simulink model "C172S_AltitudeHold_V1"  (R2026a)
settings: Solver=ode4  StartTime=0  StopTime=180  FixedStep=0.02
InitFcn:
  | ah1Data = c172sLongitudinalData();
  | [~,ah1Plant] = c172sLongitudinalPlant(ah1Data);
  | ah1PitchController = c172sPitchAttitudeControllerData();
  | ah1Actuator = c172sElevatorActuatorData();
  | ah1AltitudeController = c172sAltitudeHoldControllerData();
  | A_ah1 = ah1Plant.A; B_ah1 = ah1Plant.B;
  | C_ah1 = ah1Plant.C; D_ah1 = ah1Plant.D;
  | Vtrim_ah1_mps = ah1Data.trim.V_mps;
  | Kh_ah1_per_s = ah1AltitudeController.altitudeGain_per_s;
  | Kv_ah1_radPerMps = ah1AltitudeController.verticalSpeedGain_radPerMps;
  | tauAltitude_ah1_s = ah1AltitudeController.commandFilterTimeConstant_s;
  | hDotLimit_ah1_mps = ah1AltitudeController.verticalSpeedCommandLimit_mps;
  | thetaLimit_ah1_rad = ah1AltitudeController.pitchCommandLimit_rad;
  | Kp_ah1 = ah1PitchController.Kp_radPerRad;
  | Ki_ah1_per_s = ah1PitchController.Ki_radPerRadPerS;
  | Kq_ah1_s = ah1Actuator.integration.Kq_s;
  | tauTheta_ah1_s = ah1PitchController.commandFilterTimeConstant_s;
  | tauActuator_ah1_s = ah1Actuator.dynamics.timeConstant_s;
  | Tt_ah1_s = ah1Actuator.antiWindup.trackingTimeConstant_s;
  | deltaELower_ah1_rad = ah1Actuator.authority.lowerLimit_rad;
  | deltaEUpper_ah1_rad = ah1Actuator.authority.upperLimit_rad;
  | deltaERate_ah1_radps = deg2rad(ah1Actuator.dynamics.rateLimit_degps);
  | if ~exist('hCommand_ah1_m','var'), hCommand_ah1_m = ah1AltitudeController.validation.operationalCommand_m; end
  | if ~exist('antiWindupEnable_ah1','var'), antiWindupEnable_ah1 = 1.0; end
  | if ~exist('x0_ah1','var'), x0_ah1 = zeros(4,1); end
  | if ~exist('xi0_ah1','var'), xi0_ah1 = 0.0; end
  | if ~exist('deltaE0_ah1','var'), deltaE0_ah1 = 0.0; end
  | if ~exist('h0_ah1_m','var'), h0_ah1_m = 0.0; end
undefined symbols (not defined in the file or in its folder): antiWindupEnable_ah1, deltaE0_ah1, h0_ah1_m, x0_ah1, xi0_ah1
settings Model: Creator=Shahi  LastModifiedBy=Shahi

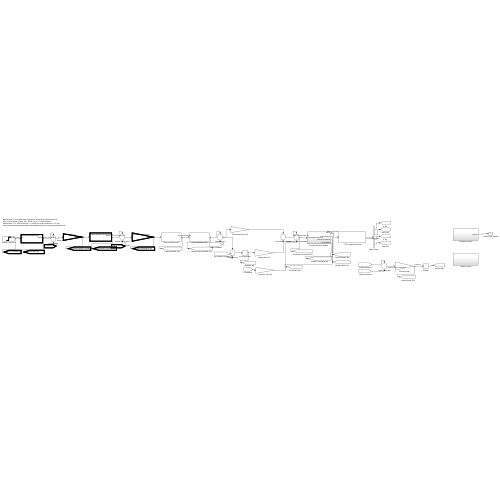
[thumbnail: Simulink's stored preview of the top-level diagram]
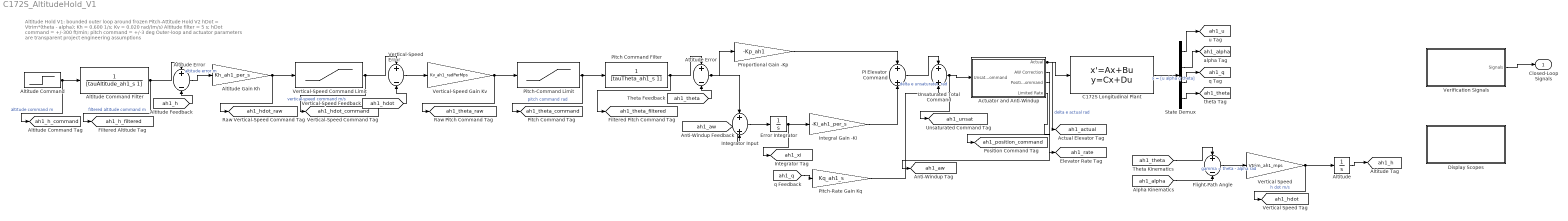
== system C172S_AltitudeHold_V1 ==
  note: Altitude Hold V1: bounded outer loop around frozen Pitch-Attitude Hold V2
      | hDot = Vtrim*(theta - alpha); Kh = 0.600 1/s; Kv = 0.020 rad/(m/s)
      | Altitude filter = 5 s; hDot command = +/-300 ft/min; pitch command = +/-3 deg
      | Outer-loop and actuator parameters are transparent project engineering assumptions
  Actuator and Anti-Windup : Subsystem
  Altitude : Integrator  InitialCondition=h0_ah1_m
  Altitude Command : Step  Time=0  FinalValue=hCommand_ah1_m  SampleTime=0
  Altitude Command Filter : TransferFcn  Numerator=1  Denominator=[tauAltitude_ah1_s 1]
  Altitude Error : Sum  Inputs=+-
  Altitude Gain Kh : Gain  Gain=Kh_ah1_per_s
  Attitude Error : Sum  Inputs=+-
  C172S Longitudinal Plant : StateSpace  A=A_ah1  B=B_ah1  C=C_ah1  D=D_ah1  InitialCondition=x0_ah1
  Display Scopes : Subsystem
  Error Integrator : Integrator  InitialCondition=xi0_ah1
  Flight-Path Angle : Sum  Inputs=+-
  Integral Gain -Ki : Gain  Gain=-Ki_ah1_per_s
  Integrator Input : Sum
  PI Elevator Command : Sum
  Pitch Command Filter : TransferFcn  Numerator=1  Denominator=[tauTheta_ah1_s 1]
  Pitch-Command Limit : Saturate  UpperLimit=thetaLimit_ah1_rad  LowerLimit=-thetaLimit_ah1_rad
  Pitch-Rate Gain Kq : Gain  Gain=Kq_ah1_s
  Proportional Gain -Kp : Gain  Gain=-Kp_ah1
  State Demux : Demux
  Unsaturated Total Command : Sum
  Verification Signals : Subsystem
  Vertical Speed : Gain  Gain=Vtrim_ah1_mps
  Vertical-Speed Command Limit : Saturate  UpperLimit=hDotLimit_ah1_mps  LowerLimit=-hDotLimit_ah1_mps
  Vertical-Speed Error : Sum  Inputs=+-
  Vertical-Speed Gain Kv : Gain  Gain=Kv_ah1_radPerMps
  Closed-Loop Signals : Outport
  tag scope: ah1_actual=global, ah1_alpha=global, ah1_aw=global, ah1_h=global, ah1_h_command=global, ah1_h_filtered=global, ah1_hdot=global, ah1_hdot_command=global, ah1_hdot_raw=global, ah1_position_command=global, ah1_q=global, ah1_rate=global, ah1_theta=global, ah1_theta_command=global, ah1_theta_filtered=global, ah1_theta_raw=global, ah1_u=global, ah1_unsat=global, ah1_xi=global
  wires:
  Altitude Command/1 -> Altitude Command Filter/1, [ah1_h_command]  "altitude command m"
  Altitude Command Filter/1 -> Altitude Error/1, [ah1_h_filtered]  "filtered altitude command m"
  [ah1_h] -> Altitude Error/2
  Altitude Error/1 -> Altitude Gain Kh/1  "altitude error m"
  Altitude Gain Kh/1 -> Vertical-Speed Command Limit/1, [ah1_hdot_raw]
  Vertical-Speed Command Limit/1 -> Vertical-Speed Error/1, [ah1_hdot_command]  "vertical-speed command m/s"
  [ah1_hdot] -> Vertical-Speed Error/2
  Vertical-Speed Error/1 -> Vertical-Speed Gain Kv/1
  Vertical-Speed Gain Kv/1 -> Pitch-Command Limit/1, [ah1_theta_raw]
  Pitch-Command Limit/1 -> Pitch Command Filter/1, [ah1_theta_command]  "pitch command rad"
  Pitch Command Filter/1 -> Attitude Error/1, [ah1_theta_filtered]
  [ah1_theta] -> Attitude Error/2
  Attitude Error/1 -> Proportional Gain -Kp/1, Integrator Input/1
  [ah1_aw] -> Integrator Input/2
  Integrator Input/1 -> Error Integrator/1
  Error Integrator/1 -> Integral Gain -Ki/1, [ah1_xi]
  Proportional Gain -Kp/1 -> PI Elevator Command/1
  Integral Gain -Ki/1 -> PI Elevator Command/2
  [ah1_q] -> Pitch-Rate Gain Kq/1
  PI Elevator Command/1 -> Unsaturated Total Command/1
  Pitch-Rate Gain Kq/1 -> Unsaturated Total Command/2
  Unsaturated Total Command/1 -> Actuator and Anti-Windup/1(Unsaturated Command), [ah1_unsat]  "delta e unsaturated rad"
  Actuator and Anti-Windup/1(Actual) -> C172S Longitudinal Plant/1, [ah1_actual]  "delta e actual rad"
  C172S Longitudinal Plant/1 -> State Demux/1  "x = [u alpha q theta]"
  [ah1_theta] -> Flight-Path Angle/1
  [ah1_alpha] -> Flight-Path Angle/2
  Flight-Path Angle/1 -> Vertical Speed/1  "gamma = theta - alpha rad"
  Vertical Speed/1 -> Altitude/1, [ah1_hdot]  "h dot m/s"
  Actuator and Anti-Windup/2(AW Correction) -> [ah1_aw]
  Actuator and Anti-Windup/3(Position Command) -> [ah1_position_command]
  Actuator and Anti-Windup/4(Limited Rate) -> [ah1_rate]
  Altitude/1 -> [ah1_h]
  State Demux/1 -> [ah1_u]
  State Demux/2 -> [ah1_alpha]
  State Demux/3 -> [ah1_q]
  State Demux/4 -> [ah1_theta]
  Verification Signals/1(Signals) -> Closed-Loop Signals/1

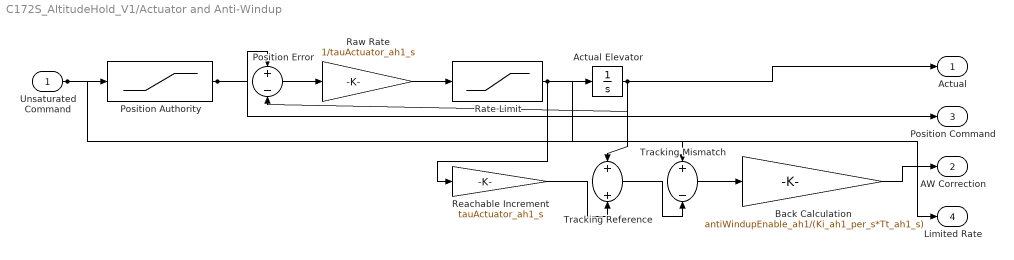
== system C172S_AltitudeHold_V1/Actuator and Anti-Windup ==
  Unsaturated Command : Inport
  Actual Elevator : Integrator  InitialCondition=deltaE0_ah1
  Back Calculation : Gain  Gain=antiWindupEnable_ah1/(Ki_ah1_per_s*Tt_ah1_s)
  Position Authority : Saturate  UpperLimit=deltaEUpper_ah1_rad  LowerLimit=deltaELower_ah1_rad
  Position Error : Sum  Inputs=+-
  Rate Limit : Saturate  UpperLimit=deltaERate_ah1_radps  LowerLimit=-deltaERate_ah1_radps
  Raw Rate : Gain  Gain=1/tauActuator_ah1_s
  Reachable Increment : Gain  Gain=tauActuator_ah1_s
  Tracking Mismatch : Sum  Inputs=+-
  Tracking Reference : Sum
  Actual : Outport
  AW Correction : Outport  Port=2
  Position Command : Outport  Port=3
  Limited Rate : Outport  Port=4
  wires:
  Unsaturated Command/1 -> Position Authority/1, Tracking Mismatch/1
  Position Authority/1 -> Position Error/1, Position Command/1
  Position Error/1 -> Raw Rate/1
  Raw Rate/1 -> Rate Limit/1
  Rate Limit/1 -> Actual Elevator/1, Reachable Increment/1, Limited Rate/1
  Actual Elevator/1 -> Position Error/2, Tracking Reference/1, Actual/1
  Reachable Increment/1 -> Tracking Reference/2
  Tracking Reference/1 -> Tracking Mismatch/2
  Tracking Mismatch/1 -> Back Calculation/1
  Back Calculation/1 -> AW Correction/1

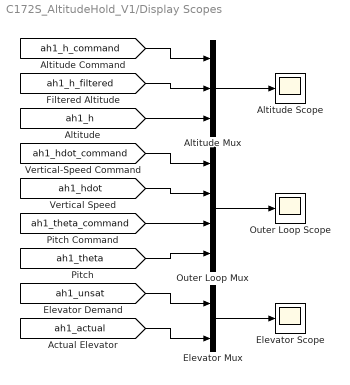
== system C172S_AltitudeHold_V1/Display Scopes ==
  Altitude Mux : Mux  Inputs=3
  Altitude Scope : Scope
  Elevator Mux : Mux  Inputs=2
  Elevator Scope : Scope
  Outer Loop Mux : Mux
  Outer Loop Scope : Scope
  wires:
  [ah1_h_command] -> Altitude Mux/1
  [ah1_h_filtered] -> Altitude Mux/2
  [ah1_h] -> Altitude Mux/3
  Altitude Mux/1 -> Altitude Scope/1
  [ah1_hdot_command] -> Outer Loop Mux/1
  [ah1_hdot] -> Outer Loop Mux/2
  [ah1_theta_command] -> Outer Loop Mux/3
  [ah1_theta] -> Outer Loop Mux/4
  Outer Loop Mux/1 -> Outer Loop Scope/1
  [ah1_unsat] -> Elevator Mux/1
  [ah1_actual] -> Elevator Mux/2
  Elevator Mux/1 -> Elevator Scope/1

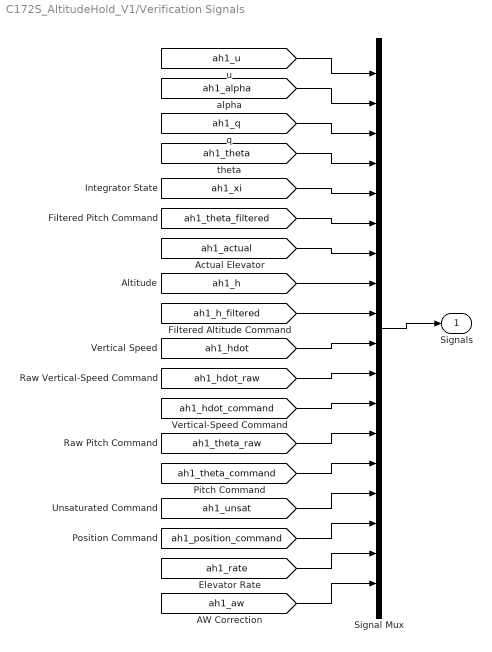
== system C172S_AltitudeHold_V1/Verification Signals ==
  Signal Mux : Mux  Inputs=18
  Signals : Outport
  wires:
  [ah1_u] -> Signal Mux/1
  [ah1_alpha] -> Signal Mux/2
  [ah1_q] -> Signal Mux/3
  [ah1_theta] -> Signal Mux/4
  [ah1_xi] -> Signal Mux/5
  [ah1_theta_filtered] -> Signal Mux/6
  [ah1_actual] -> Signal Mux/7
  [ah1_h] -> Signal Mux/8
  [ah1_h_filtered] -> Signal Mux/9
  [ah1_hdot] -> Signal Mux/10
  [ah1_hdot_raw] -> Signal Mux/11
  [ah1_hdot_command] -> Signal Mux/12
  [ah1_theta_raw] -> Signal Mux/13
  [ah1_theta_command] -> Signal Mux/14
  [ah1_unsat] -> Signal Mux/15
  [ah1_position_command] -> Signal Mux/16
  [ah1_rate] -> Signal Mux/17
  [ah1_aw] -> Signal Mux/18
  Signal Mux/1 -> Signals/1
